simulink model "threePHASE_INVERTER_SPWM"  (R2023a)
settings: Solver=VariableStepAuto  StartTime=0.0  StopTime=10.0  RelTol=1e-3
libraries: spsMosfetLib x6, simulink x3, spsDCVoltageSourceLib x1, spsGroundLib x1, spsSawtoothGeneratorLib x1, spsThreePhaseSeriesRLCBranchLib x1, spsThreePhaseVIMeasurementLib x1, spspowerguiLib x1
settings Model: Creator=Ganesh Fashion  LastModifiedBy=Ganesh Fashion

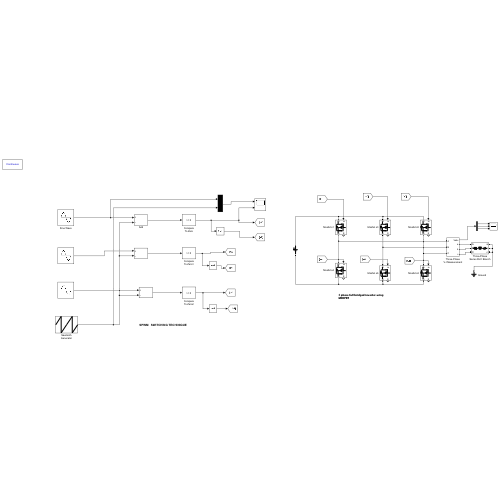
[thumbnail: Simulink's stored preview of the top-level diagram]
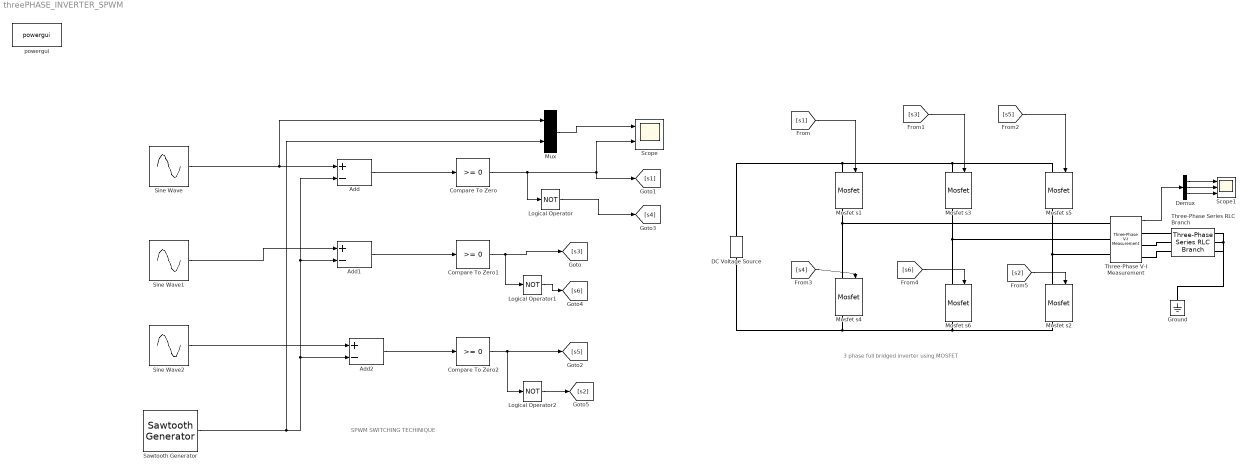
== system threePHASE_INVERTER_SPWM ==
  note: SPWM SWITCHING TECHINIQUE
  note: 3 phase full bridged inverter using MOSFET
  Add : Sum  Inputs=+-
  Add1 : Sum  Inputs=+-
  Add2 : Sum  Inputs=+-
  Compare To Zero : simulink/Logic and Bit Operations/Compare To Zero  relop=>=  OutDataTypeStr=boolean
  Compare To Zero1 : simulink/Logic and Bit Operations/Compare To Zero  relop=>=  OutDataTypeStr=boolean
  Compare To Zero2 : simulink/Logic and Bit Operations/Compare To Zero  relop=>=  OutDataTypeStr=boolean
  DC Voltage Source : spsDCVoltageSourceLib/DC Voltage Source  Amplitude=100  Measurements=None
  Demux : Demux  Outputs=3
  Ground : spsGroundLib/Ground  LConnTagsString=a
  Logical Operator : Logic  Operator=NOT  AllPortsSameDT=off  OutDataTypeStr=boolean
  Logical Operator1 : Logic  Operator=NOT  AllPortsSameDT=off  OutDataTypeStr=boolean
  Logical Operator2 : Logic  Operator=NOT  AllPortsSameDT=off  OutDataTypeStr=boolean
  Mosfet s{1..6} (6 alike) : spsMosfetLib/Mosfet  Ron=0.1  Lon=0  Rd=0.01  Vfd=0  IC=0  Rs=1e5  Cs=inf  Measurements=on
  Mux : Mux  Inputs=2
  Sawtooth Generator : spsSawtoothGeneratorLib/Sawtooth Generator  Freq=1e3  Phase=180  Ts=0
  Scope : Scope  NumInputPorts=2
  Scope1 : Scope  NumInputPorts=3
  Sine Wave : Sin  Frequency=2*pi*50  SampleTime=0
  Sine Wave1 : Sin  Frequency=2*pi*50  Phase=2*pi/3  SampleTime=0
  Sine Wave2 : Sin  Frequency=2*pi*50  Phase=4*pi/3  SampleTime=0
  Three-Phase Series RLC Branch : spsThreePhaseSeriesRLCBranchLib/Three-Phase Series RLC Branch  LConnTagsString=A|B|C  RConnTagsString=A|B|C  BranchType=RLC  Resistance=1  Inductance=1e-3  Capacitance=1e-6  Measurements=None
  Three-Phase V-I Measurement : spsThreePhaseVIMeasurementLib/Three-Phase V-I Measurement  VoltageMeasurement=phase-to-ground  SetLabelV=off  LabelV=Vabc  Vpu=off  VpuLL=off  CurrentMeasurement=no  SetLabelI=off  LabelI=Iabc  Ipu=off  Pbase=100e6  Vbase=500e3  OutputType=Complex  PhasorSimulation=off  PSBequivalent=0
  powergui : spspowerguiLib/powergui  Priority=1  SimulationMode=Continuous  SampleTime=50e-6  frequency=60  Iterations=50  frequencyindice=0  Pbase=100e6  ErrMax=1e-4  UnitsV=kV  UnitsW=MW  buscounter=0  FunctionMessages=off  echomessages=off  EnableUseOfTLC=off  CurrentSourceSwitches=off  DisableSnubberDevices=off  DisableRonSwitches=off  DisableVfSwitches=off  DisplayEquations=off  AutomaticDiscreteSolvers=off  SolverType=Tustin/Backward Euler (TBE)  Interpol=off  ExternalGateDelay=off  methode=off  Ts=100  x0status=blocks  SPID=on  SwTol=0  HookPort=off  NonlinearTolerance=1e-4  nMaxIteration=100  ContinueOnMaxIteration=off  RestoreLinks=warning  ResistiveCurrentMeasurement=off  Frange=[0:2:500]  Ylog=off  Xlog=on  ShowGrid=off  save=off  variable=ZData  structure=0  ZoomFFT=off  StartTime=0.0  cycles=1  DisplayStyle=1  fundamental=60  FreqAxis=off  MaxFrequency=1000  frequencyindicesteady=1  RmsSteady=1  display=off
  wires:
  Sine Wave/1 -> Mux/1, Add/1
  Sine Wave1/1 -> Add1/1
  Sine Wave2/1 -> Add2/1
  Sawtooth Generator/1 -> Mux/2, Add2/2, Add1/2, Add/2
  Add/1 -> Compare To Zero/1
  Add1/1 -> Compare To Zero1/1
  Add2/1 -> Compare To Zero2/1
  Compare To Zero/1 -> Logical Operator/1, Scope/2, [s1]
  Mux/1 -> Scope/1
  Compare To Zero1/1 -> Logical Operator1/1, [s3]
  Compare To Zero2/1 -> Logical Operator2/1, [s5]
  Logical Operator/1 -> [s4]
  Logical Operator1/1 -> [s6]
  Logical Operator2/1 -> [s2]
  [s1] -> Mosfet s1/1
  [s5] -> Mosfet s5/1
  [s3] -> Mosfet s3/1
  [s4] -> Mosfet s4/1
  [s6] -> Mosfet s6/1
  [s2] -> Mosfet s2/1
  Three-Phase V-I Measurement/1 -> Demux/1
  Demux/1 -> Scope1/1
  Demux/2 -> Scope1/2
  Demux/3 -> Scope1/3
  connections:
  Mosfet s1/LConn1 -- DC Voltage Source/RConn1 -- Mosfet s5/LConn1 -- Mosfet s3/LConn1
  Mosfet s1/RConn1 -- Three-Phase V-I Measurement/LConn1 -- Mosfet s4/LConn1
  Mosfet s4/RConn1 -- DC Voltage Source/LConn1 -- Mosfet s2/RConn1 -- Mosfet s6/RConn1
  Mosfet s2/LConn1 -- Three-Phase V-I Measurement/LConn3 -- Mosfet s5/RConn1
  Mosfet s6/LConn1 -- Three-Phase V-I Measurement/LConn2 -- Mosfet s3/RConn1
  Three-Phase Series RLC Branch/RConn1 -- Ground/LConn1 -- Three-Phase Series RLC Branch/RConn3 -- Three-Phase Series RLC Branch/RConn2
  Three-Phase Series RLC Branch/LConn1 -- Three-Phase V-I Measurement/RConn1
  Three-Phase Series RLC Branch/LConn2 -- Three-Phase V-I Measurement/RConn2
  Three-Phase Series RLC Branch/LConn3 -- Three-Phase V-I Measurement/RConn3
